simulink model "FMUCTRL"  (R2020b)
settings: Solver=FixedStepAuto  StartTime=0.0  StopTime=31622400  FixedStep=60  RelTol=1e-3
libraries: neural x5
settings Model: Creator=khfa  LastModifiedBy=khfa

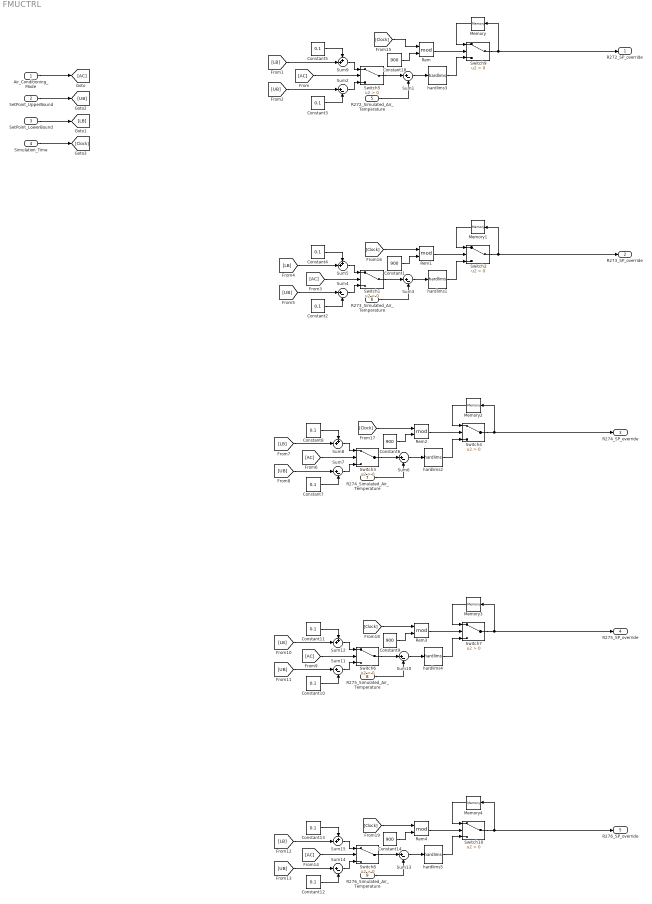
== system FMUCTRL ==
  Air_Conditioning_Mode : Inport
  SetPoint_UpperBound : Inport  Port=2
  SetPoint_LowerBound : Inport  Port=3
  Simulation_Time : Inport  Port=4
  R272_Simulated_Air_Temperature : Inport  Port=5
  R273_Simulated_Air_Temperature : Inport  Port=6
  R274_Simulated_Air_Temperature : Inport  Port=7
  R275_Simulated_Air_Temperature : Inport  Port=8
  R276_Simulated_Air_Temperature : Inport  Port=9
  Constant{1,6,9,14,18} (5 alike) : Constant  Value=900
  Constant{2..5,7..8,10..13} (10 alike) : Constant  Value=0.1
  Memory{,1..4} (5 alike) : Memory  InitialCondition=22
  Rem{,1..4} (5 alike) : Math  Operator=mod  OutputSignalType=real  SaturateOnIntegerOverflow=on
  Sum{1..4,6..7,10..11,13..14} (10 alike) : Sum  Inputs=|+-
  Sum{5,8..9,12,15} (5 alike) : Sum  Inputs=++|
  Switch{1..10} (10 alike) : Switch  Criteria=u2 > Threshold
  hardlims1 : neural/Transfer Functions/hardlims
      link override Constant: Value=32
      link override Constant1: Value=12
      settings: SourceProductBaseCode=NN
  hardlims2 : neural/Transfer Functions/hardlims
      link override Constant: Value=32
      link override Constant1: Value=12
      settings: SourceProductBaseCode=NN
  hardlims3 : neural/Transfer Functions/hardlims
      link override Constant: Value=32
      link override Constant1: Value=12
      settings: SourceProductBaseCode=NN
  hardlims4 : neural/Transfer Functions/hardlims
      link override Constant: Value=32
      link override Constant1: Value=12
      settings: SourceProductBaseCode=NN
  hardlims5 : neural/Transfer Functions/hardlims
      link override Constant: Value=32
      link override Constant1: Value=12
      settings: SourceProductBaseCode=NN
  R272_SP_override : Outport
  R273_SP_override : Outport  Port=2
  R274_SP_override : Outport  Port=3
  R275_SP_override : Outport  Port=4
  R276_SP_override : Outport  Port=5
  wires:
  Constant18/1 -> Rem/2
  Memory/1 -> Switch9/1
  Switch9/1 -> Memory/1, R272_SP_override/1
  hardlims3/1 -> Switch9/3
  Rem/1 -> Switch9/2
  Constant5/1 -> Sum9/1
  SetPoint_LowerBound/1 -> [LB]
  Sum2/1 -> Switch5/3
  R272_Simulated_Air_Temperature/1 -> Sum1/2
  Sum9/1 -> Switch5/1
  Air_Conditioning_Mode/1 -> [AC]
  Constant3/1 -> Sum2/2
  Sum1/1 -> hardlims3/1
  Switch5/1 -> Sum1/1
  Sum4/1 -> Switch1/3
  Constant1/1 -> Rem1/2
  Switch1/1 -> Sum3/1
  hardlims1/1 -> Switch2/3
  Memory1/1 -> Switch2/1
  Constant4/1 -> Sum5/1
  Sum3/1 -> hardlims1/1
  Switch2/1 -> R273_SP_override/1, Memory1/1
  Constant2/1 -> Sum4/2
  Rem1/1 -> Switch2/2
  Sum5/1 -> Switch1/1
  R273_Simulated_Air_Temperature/1 -> Sum3/2
  [Clock] -> Rem1/1
  [AC] -> Switch5/2
  [LB] -> Sum9/2
  SetPoint_UpperBound/1 -> [UB]
  [UB] -> Sum2/1
  [LB] -> Sum5/2
  [AC] -> Switch1/2
  [UB] -> Sum4/1
  [UB] -> Sum7/1
  hardlims2/1 -> Switch4/3
  Sum7/1 -> Switch3/3
  Memory2/1 -> Switch4/1
  Sum6/1 -> hardlims2/1
  Constant6/1 -> Rem2/2
  Sum8/1 -> Switch3/1
  [AC] -> Switch3/2
  Constant8/1 -> Sum8/1
  R274_Simulated_Air_Temperature/1 -> Sum6/2
  [Clock] -> Rem2/1
  Constant7/1 -> Sum7/2
  Switch4/1 -> R274_SP_override/1, Memory2/1
  [LB] -> Sum8/2
  Rem2/1 -> Switch4/2
  Switch3/1 -> Sum6/1
  Switch6/1 -> Sum10/1
  Rem3/1 -> Switch7/2
  Switch7/1 -> R275_SP_override/1, Memory3/1
  [LB] -> Sum12/2
  Constant10/1 -> Sum11/2
  Sum10/1 -> hardlims4/1
  Memory3/1 -> Switch7/1
  R275_Simulated_Air_Temperature/1 -> Sum10/2
  [Clock] -> Rem3/1
  [AC] -> Switch6/2
  Sum12/1 -> Switch6/1
  Constant9/1 -> Rem3/2
  Sum11/1 -> Switch6/3
  Constant11/1 -> Sum12/1
  hardlims4/1 -> Switch7/3
  [UB] -> Sum11/1
  R276_Simulated_Air_Temperature/1 -> Sum13/2
  Sum13/1 -> hardlims5/1
  Constant12/1 -> Sum14/2
  Switch10/1 -> R276_SP_override/1, Memory4/1
  [Clock] -> Rem4/1
  [LB] -> Sum15/2
  Rem4/1 -> Switch10/2
  Switch8/1 -> Sum13/1
  Memory4/1 -> Switch10/1
  Sum14/1 -> Switch8/3
  Constant14/1 -> Rem4/2
  Sum15/1 -> Switch8/1
  [UB] -> Sum14/1
  [AC] -> Switch8/2
  hardlims5/1 -> Switch10/3
  Constant13/1 -> Sum15/1
  Simulation_Time/1 -> [Clock]
  [Clock] -> Rem/1
